simulink model "two_link_control"  (R2025a)
settings: Solver=ode5  StartTime=0.0  StopTime=10.0  FixedStep=1e-5  RelTol=1e-3
settings Model: Creator=Lenovo  LastModifiedBy=Lenovo

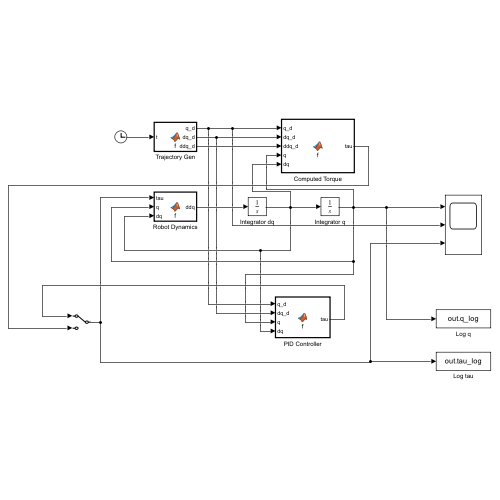
[thumbnail: Simulink's stored preview of the top-level diagram]
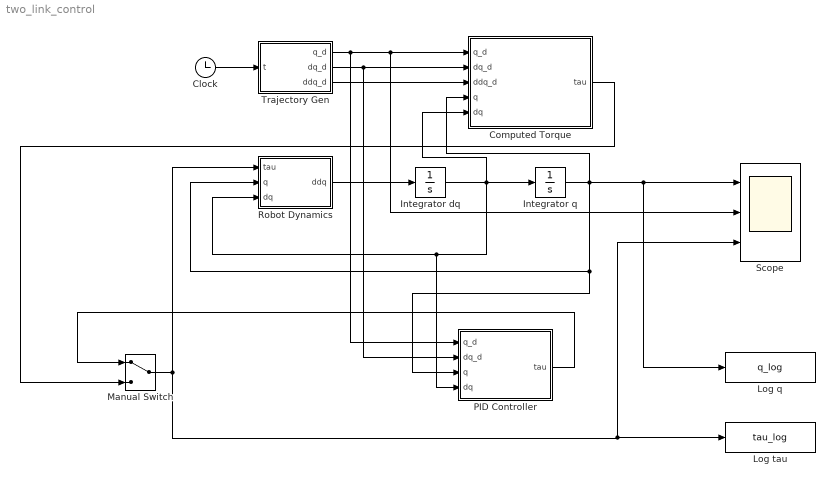
== system two_link_control ==
  Clock : Clock
  Computed Torque : MATLAB Function  TreatAsAtomicUnit=on
  Integrator dq : Integrator  InitialCondition=[-0.1; -0.05]
  Integrator q : Integrator  InitialCondition=[0;0]
  Log q : ToWorkspace  VariableName=q_log  SaveFormat=Timeseries  SampleTime=-1
  Log tau : ToWorkspace  VariableName=tau_log  SaveFormat=Timeseries  SampleTime=-1
  Manual Switch : ManualSwitch
  PID Controller : MATLAB Function  TreatAsAtomicUnit=on
  Robot Dynamics : MATLAB Function  TreatAsAtomicUnit=on
  Scope : Scope  NumInputPorts=3
      settings: ActiveDisplayYMinimum=-37040.726540590083  ActiveDisplayYMaximum=113761.52716461988
  Trajectory Gen : MATLAB Function  TreatAsAtomicUnit=on
  wires:
  Robot Dynamics/1(ddq) -> Integrator dq/1
  Integrator dq/1 -> PID Controller/4(dq), Robot Dynamics/3(dq), Computed Torque/5(dq), Integrator q/1
  Integrator q/1 -> PID Controller/3(q), Robot Dynamics/2(q), Log q/1, Scope/1, Computed Torque/4(q)
  Clock/1 -> Trajectory Gen/1(t)
  Trajectory Gen/1(q_d) -> Scope/2, Computed Torque/1(q_d), PID Controller/1(q_d)
  Trajectory Gen/2(dq_d) -> PID Controller/2(dq_d), Computed Torque/2(dq_d)
  Trajectory Gen/3(ddq_d) -> Computed Torque/3(ddq_d)
  Manual Switch/1 -> Robot Dynamics/1(tau), Log tau/1, Scope/3
  Computed Torque/1(tau) -> Manual Switch/2
  PID Controller/1(tau) -> Manual Switch/1

== matlab function two_link_control/Trajectory Gen ==
  data: t input; q_d output; dq_d output; ddq_d output
function [q_d, dq_d, ddq_d] = f(t)
q_d = [sin(2*t); 0.5*sin(3*t)];
dq_d = [2*cos(2*t); 1.5*cos(3*t)];
ddq_d = [-4*sin(2*t); -4.5*sin(3*t)];

== matlab function two_link_control/Robot Dynamics ==
  data: tau input; ddq output; q input; dq input
function ddq = f(tau, q, dq)
l1=1.0; l2=0.8; m1=10; m2=5; I1=0.83; I2=0.21; g=9.81;
c2=cos(q(2)); s2=sin(q(2));
M11=I1+I2+m1*l1^2/4+m2*(l1^2+l2^2/4+l1*l2*c2);
M12=I2+m2*(l2^2/4+l1*l2*c2/2);
M22=I2+m2*l2^2/4;
M=[M11,M12;M12,M22];
h=-m2*l1*l2*s2/2;
C=[h*dq(2)*(2*dq(1)+dq(2)); h*dq(1)^2];
G=[g*cos(q(1))*(m1*l1/2+m2*l1)+g*m2*l2*cos(q(1)+q(2))/2; g*m2*l2*cos(q(1)+q(2))/2];
ddq = M \ (tau - C - G);

== matlab function two_link_control/Computed Torque ==
  data: q_d input; tau output; dq_d input; ddq_d input; q input; dq input
function tau = f(q_d, dq_d, ddq_d, q, dq)
l1=1.0; l2=0.8; m1=10; m2=5; I1=0.83; I2=0.21; g=9.81;
c2=cos(q(2)); s2=sin(q(2));
M11=I1+I2+m1*l1^2/4+m2*(l1^2+l2^2/4+l1*l2*c2);
M12=I2+m2*(l2^2/4+l1*l2*c2/2);
M22=I2+m2*l2^2/4;
M=[M11,M12;M12,M22];
h=-m2*l1*l2*s2/2;
C=[h*dq(2)*(2*dq(1)+dq(2)); h*dq(1)^2];
G=[g*cos(q(1))*(m1*l1/2+m2*l1)+g*m2*l2*cos(q(1)+q(2))/2; g*m2*l2*cos(q(1)+q(2))/2];
e=q_d-q; de=dq_d-dq;
Kp=[100;80]; Kd=[30;25];
tau = M*(ddq_d + Kp.*e + Kd.*de) + C + G;

== matlab function two_link_control/PID Controller ==
  settings: updateMethod=DISCRETE
  data: q_d input; tau output; dq_d input; q input; dq input
function tau = f(q_d, dq_d, q, dq)
Kp=[800;600]; Ki=[50;30]; Kd=[100;80];
persistent int_e
if isempty(int_e), int_e=[0;0]; end
e = q_d - q;
de = dq_d - dq;
int_e = int_e + e * 0.01;  % dt=0.01
int_e = max(min(int_e, 10), -10);  % 抗饱和
tau = Kp.*e + Ki.*int_e + Kd.*de;
